simulink model "Channelizer_smoke"  (R2025a)
settings: Solver=VariableStepAuto  StartTime=0.0  StopTime=8359  RelTol=1e-3
PostLoadFcn:
  | gen_coeffs;
InitFcn:
  | gen_coeffs;
values from neighbouring files (symbols this model uses):
  coeff_matrix = zeros([num_fir_units, default_num_chan, fir_taps])    [coeffs_for_fir_units.m]    (also in gen_coeffs.m = squeeze(coeffs_for_fir_units(prototype_fir, config))')
undefined symbols (not defined in the file or in its folder): dspblkCoreblockFVToolHelper, es1, gcbh, S, vsva2488, xcvr1602
libraries: hdlBasic x27, dspsrcs4 x17, hdlDSPIP x1, vmcUtilities x1
settings Model: Creator=nanumolu  LastModifiedBy=robg

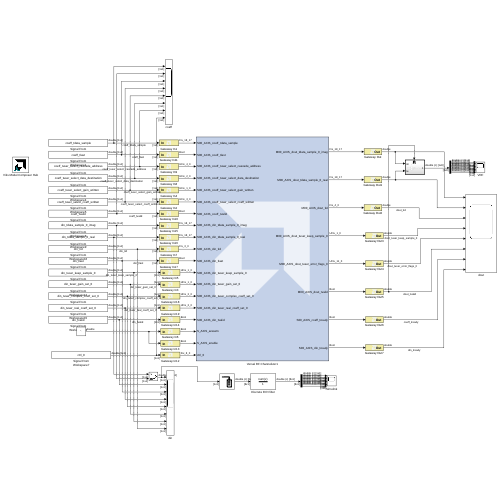
[thumbnail: Simulink's stored preview of the top-level diagram]
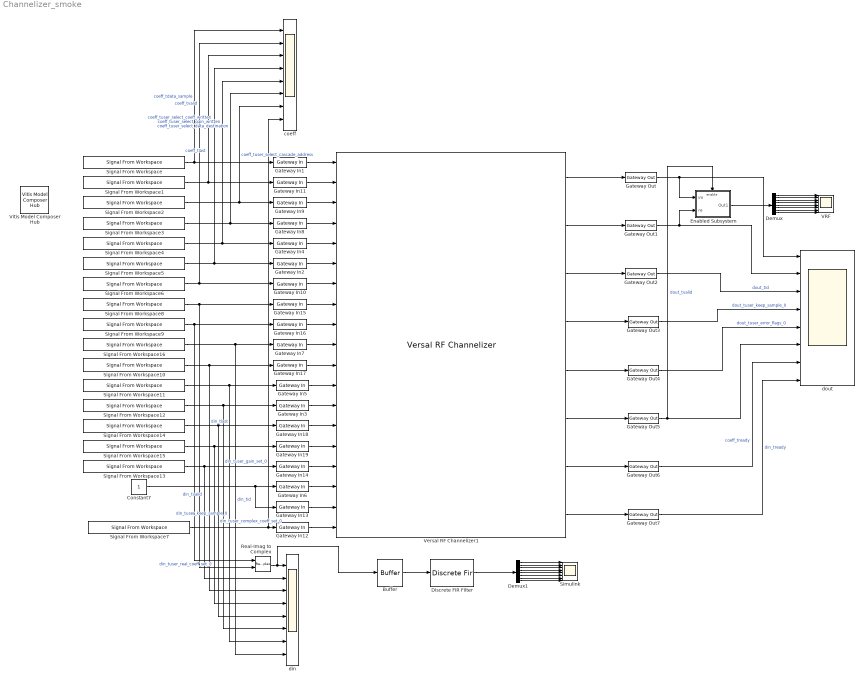
== system Channelizer_smoke ==
  Buffer : Buffer  N=8  OutputFrames=off
  Constant7 : Constant
  Demux : Demux  Outputs=8
  Demux1 : Demux  Outputs=8
  Discrete FIR Filter : DiscreteFir  LoadFcn=dspblkCoreblockFVToolHelper(gcbh,'load');  Coefficients=coeff_matrix(:,1)'  InputProcessing=Columns as channels (frame based)
      settings: CopyFcn=dspblkCoreblockFVToolHelper(gcbh,'copy');  DeleteFcn=dspblkCoreblockFVToolHelper(gcbh,'close');  ModelCloseFcn=dspblkCoreblockFVToolHelper(gcbh,'close');  PreSaveFcn=dspblkCoreblockFVToolHelper(gcbh,'presave');  PostSaveFcn=dspblkCoreblockFVToolHelper(gcbh,'postsave');  CloseFcn=dspblkCoreblockFVToolHelper(gcbh,'close');
  Enabled Subsystem : Subsystem  TreatAsAtomicUnit=on
  Gateway In1 : hdlBasic/Gateway In  gui_display_data_type=Fixed-point  arith_type=Signed (2's comp)  n_bits=18  bin_pt=17  preci_type=Single  exp_width=8  frac_width=24  rows=1  columns=1  quantization="Round  (unbiased: +/- Inf)"  overflow=Saturate  period=1  UseAsADC=off  ADCChannel='1'  interface=None  automatic_assignment=on  address_offset=hex2dec('00')  intf_name=''  intf_description=''  default_value=0  timing_constraint=None  locs_specified=off  LOCs={}  io_standard={}  inherit_from_input=off  hdl_port=on  XmcBlockStatus=1  maskContainerNames=group4  block_type=gatewayin  block_config=sysgen:gateway_in_config  block_width_w=590  block_height_w=620  block_width=640  block_height=850
  Gateway In{6,10..11,13..14,17} (6 alike) : hdlBasic/Gateway In  gui_display_data_type=Boolean  arith_type=Boolean  n_bits=16  bin_pt=14  preci_type=Single  exp_width=8  frac_width=24  rows=1  columns=1  quantization="Round  (unbiased: +/- Inf)"  overflow=Saturate  period=1  UseAsADC=off  ADCChannel='1'  interface=None  automatic_assignment=on  address_offset=hex2dec('00')  intf_name=''  intf_description=''  default_value=0  timing_constraint=None  locs_specified=off  LOCs={}  io_standard={}  inherit_from_input=off  hdl_port=on  XmcBlockStatus=1  maskContainerNames=group4  block_type=gatewayin  block_config=sysgen:gateway_in_config  block_width_w=590  block_height_w=620  block_width=640  block_height=850
  Gateway In12 : hdlBasic/Gateway In  gui_display_data_type=Fixed-point  arith_type=Signed (2's comp)  n_bits=8  bin_pt=0  preci_type=Single  exp_width=8  frac_width=24  rows=1  columns=1  quantization="Round  (unbiased: +/- Inf)"  overflow=Saturate  period=1  UseAsADC=off  ADCChannel='1'  interface=None  automatic_assignment=on  address_offset=hex2dec('00')  intf_name=''  intf_description=''  default_value=0  timing_constraint=None  locs_specified=off  LOCs={}  io_standard={}  inherit_from_input=off  hdl_port=on  XmcBlockStatus=1  maskContainerNames=group4  block_type=gatewayin  block_config=sysgen:gateway_in_config  block_width_w=590  block_height_w=620  block_width=640  block_height=850
  Gateway In15 : hdlBasic/Gateway In  gui_display_data_type=Fixed-point  arith_type=Signed (2's comp)  n_bits=18  bin_pt=17  preci_type=Single  exp_width=8  frac_width=24  rows=1  columns=1  quantization="Round  (unbiased: +/- Inf)"  overflow=Saturate  period=1  UseAsADC=off  ADCChannel='1'  interface=None  automatic_assignment=on  address_offset=hex2dec('00')  intf_name=''  intf_description=''  default_value=0  timing_constraint=None  locs_specified=off  LOCs={}  io_standard={}  inherit_from_input=off  hdl_port=on  XmcBlockStatus=1  maskContainerNames=group4  block_type=gatewayin  block_config=sysgen:gateway_in_config  block_width_w=590  block_height_w=620  block_width=640  block_height=850
  Gateway In16 : hdlBasic/Gateway In  gui_display_data_type=Fixed-point  arith_type=Signed (2's comp)  n_bits=18  bin_pt=17  preci_type=Single  exp_width=8  frac_width=24  rows=1  columns=1  quantization="Round  (unbiased: +/- Inf)"  overflow=Saturate  period=1  UseAsADC=off  ADCChannel='1'  interface=None  automatic_assignment=on  address_offset=hex2dec('00')  intf_name=''  intf_description=''  default_value=0  timing_constraint=None  locs_specified=off  LOCs={}  io_standard={}  inherit_from_input=off  hdl_port=on  XmcBlockStatus=1  maskContainerNames=group4  block_type=gatewayin  block_config=sysgen:gateway_in_config  block_width_w=590  block_height_w=620  block_width=640  block_height=850
  Gateway In18 : hdlBasic/Gateway In  gui_display_data_type=Fixed-point  arith_type=Unsigned  n_bits=3  bin_pt=0  preci_type=Single  exp_width=8  frac_width=24  rows=1  columns=1  quantization="Round  (unbiased: +/- Inf)"  overflow=Saturate  period=1  UseAsADC=off  ADCChannel='1'  interface=None  automatic_assignment=on  address_offset=hex2dec('00')  intf_name=''  intf_description=''  default_value=0  timing_constraint=None  locs_specified=off  LOCs={}  io_standard={}  inherit_from_input=off  hdl_port=on  XmcBlockStatus=1  maskContainerNames=group4  block_type=gatewayin  block_config=sysgen:gateway_in_config  block_width_w=590  block_height_w=620  block_width=640  block_height=850
  Gateway In19 : hdlBasic/Gateway In  gui_display_data_type=Fixed-point  arith_type=Unsigned  n_bits=3  bin_pt=0  preci_type=Single  exp_width=8  frac_width=24  rows=1  columns=1  quantization="Round  (unbiased: +/- Inf)"  overflow=Saturate  period=1  UseAsADC=off  ADCChannel='1'  interface=None  automatic_assignment=on  address_offset=hex2dec('00')  intf_name=''  intf_description=''  default_value=0  timing_constraint=None  locs_specified=off  LOCs={}  io_standard={}  inherit_from_input=off  hdl_port=on  XmcBlockStatus=1  maskContainerNames=group4  block_type=gatewayin  block_config=sysgen:gateway_in_config  block_width_w=590  block_height_w=620  block_width=640  block_height=850
  Gateway In2 : hdlBasic/Gateway In  gui_display_data_type=Fixed-point  arith_type=Unsigned  n_bits=3  bin_pt=0  preci_type=Single  exp_width=8  frac_width=24  rows=1  columns=1  quantization="Round  (unbiased: +/- Inf)"  overflow=Saturate  period=1  UseAsADC=off  ADCChannel='1'  interface=None  automatic_assignment=on  address_offset=hex2dec('00')  intf_name=''  intf_description=''  default_value=0  timing_constraint=None  locs_specified=off  LOCs={}  io_standard={}  inherit_from_input=off  hdl_port=on  XmcBlockStatus=1  maskContainerNames=group4  block_type=gatewayin  block_config=sysgen:gateway_in_config  block_width_w=590  block_height_w=620  block_width=640  block_height=850
  Gateway In3 : hdlBasic/Gateway In  gui_display_data_type=Fixed-point  arith_type=Unsigned  n_bits=1  bin_pt=0  preci_type=Single  exp_width=8  frac_width=24  rows=1  columns=1  quantization="Round  (unbiased: +/- Inf)"  overflow=Saturate  period=1  UseAsADC=off  ADCChannel='1'  interface=None  automatic_assignment=on  address_offset=hex2dec('00')  intf_name=''  intf_description=''  default_value=0  timing_constraint=None  locs_specified=off  LOCs={}  io_standard={}  inherit_from_input=off  hdl_port=on  XmcBlockStatus=1  maskContainerNames=group4  block_type=gatewayin  block_config=sysgen:gateway_in_config  block_width_w=590  block_height_w=620  block_width=640  block_height=850
  Gateway In4 : hdlBasic/Gateway In  gui_display_data_type=Fixed-point  arith_type=Unsigned  n_bits=1  bin_pt=0  preci_type=Single  exp_width=8  frac_width=24  rows=1  columns=1  quantization="Round  (unbiased: +/- Inf)"  overflow=Saturate  period=1  UseAsADC=off  ADCChannel='1'  interface=None  automatic_assignment=on  address_offset=hex2dec('00')  intf_name=''  intf_description=''  default_value=0  timing_constraint=None  locs_specified=off  LOCs={}  io_standard={}  inherit_from_input=off  hdl_port=on  XmcBlockStatus=1  maskContainerNames=group4  block_type=gatewayin  block_config=sysgen:gateway_in_config  block_width_w=590  block_height_w=620  block_width=640  block_height=850
  Gateway In5 : hdlBasic/Gateway In  gui_display_data_type=Fixed-point  arith_type=Unsigned  n_bits=1  bin_pt=0  preci_type=Single  exp_width=8  frac_width=24  rows=1  columns=1  quantization="Round  (unbiased: +/- Inf)"  overflow=Saturate  period=1  UseAsADC=off  ADCChannel='1'  interface=None  automatic_assignment=on  address_offset=hex2dec('00')  intf_name=''  intf_description=''  default_value=0  timing_constraint=None  locs_specified=off  LOCs={}  io_standard={}  inherit_from_input=off  hdl_port=on  XmcBlockStatus=1  maskContainerNames=group4  block_type=gatewayin  block_config=sysgen:gateway_in_config  block_width_w=590  block_height_w=620  block_width=640  block_height=850
  Gateway In7 : hdlBasic/Gateway In  gui_display_data_type=Fixed-point  arith_type=Signed (2's comp)  n_bits=3  bin_pt=0  preci_type=Single  exp_width=8  frac_width=24  rows=1  columns=1  quantization="Round  (unbiased: +/- Inf)"  overflow=Saturate  period=1  UseAsADC=off  ADCChannel='1'  interface=None  automatic_assignment=on  address_offset=hex2dec('00')  intf_name=''  intf_description=''  default_value=0  timing_constraint=None  locs_specified=off  LOCs={}  io_standard={}  inherit_from_input=off  hdl_port=on  XmcBlockStatus=1  maskContainerNames=group4  block_type=gatewayin  block_config=sysgen:gateway_in_config  block_width_w=590  block_height_w=620  block_width=640  block_height=850
  Gateway In8 : hdlBasic/Gateway In  gui_display_data_type=Fixed-point  arith_type=Unsigned  n_bits=2  bin_pt=0  preci_type=Single  exp_width=8  frac_width=24  rows=1  columns=1  quantization="Round  (unbiased: +/- Inf)"  overflow=Saturate  period=1  UseAsADC=off  ADCChannel='1'  interface=None  automatic_assignment=on  address_offset=hex2dec('00')  intf_name=''  intf_description=''  default_value=0  timing_constraint=None  locs_specified=off  LOCs={}  io_standard={}  inherit_from_input=off  hdl_port=on  XmcBlockStatus=1  maskContainerNames=group4  block_type=gatewayin  block_config=sysgen:gateway_in_config  block_width_w=590  block_height_w=620  block_width=640  block_height=850
  Gateway In9 : hdlBasic/Gateway In  gui_display_data_type=Fixed-point  arith_type=Unsigned  n_bits=4  bin_pt=0  preci_type=Single  exp_width=8  frac_width=24  rows=1  columns=1  quantization="Round  (unbiased: +/- Inf)"  overflow=Saturate  period=1  UseAsADC=off  ADCChannel='1'  interface=None  automatic_assignment=on  address_offset=hex2dec('00')  intf_name=''  intf_description=''  default_value=0  timing_constraint=None  locs_specified=off  LOCs={}  io_standard={}  inherit_from_input=off  hdl_port=on  XmcBlockStatus=1  maskContainerNames=group4  block_type=gatewayin  block_config=sysgen:gateway_in_config  block_width_w=590  block_height_w=620  block_width=640  block_height=850
  Gateway Out{,1..7} (8 alike) : hdlBasic/Gateway Out  inherit_from_input=off  bool_to_boolean=off  hdl_port=on  rows=1  columns=1  UseAsDAC=off  DACChannel='1'  interface=None  automatic_assignment=on  address_offset=hex2dec('00')  intf_name=''  intf_description=''  timing_constraint=None  locs_specified=off  LOCs={}  io_standard={}  XmcBlockStatus=1  maskContainerNames=group4  block_type=gatewayout  block_config=sysgen:gateway_out_config  block_width_w=590  block_height_w=620  block_width=620  block_height=750
  Real-Imag to Complex : RealImagToComplex
  Signal From Workspace : dspsrcs4/Signal From Workspace  X=coeff_tdata_sample  Ts=1  nsamps=1  OutputAfterFinalValue=Setting to zero  ignoreOrWarnInputAndFrameLengths=off  OutputFrames=off
  Signal From Workspace1 : dspsrcs4/Signal From Workspace  X=coeff_tlast  Ts=1  nsamps=1  OutputAfterFinalValue=Setting to zero  ignoreOrWarnInputAndFrameLengths=off  OutputFrames=off
  Signal From Workspace10 : dspsrcs4/Signal From Workspace  X=din_tlast  Ts=1  nsamps=1  OutputAfterFinalValue=Setting to zero  ignoreOrWarnInputAndFrameLengths=off  OutputFrames=off
  Signal From Workspace11 : dspsrcs4/Signal From Workspace  X=din_tuser_keep_sample_0  Ts=1  nsamps=1  OutputAfterFinalValue=Setting to zero  ignoreOrWarnInputAndFrameLengths=off  OutputFrames=off
  Signal From Workspace12 : dspsrcs4/Signal From Workspace  X=din_tuser_gain_set_0  Ts=1  nsamps=1  OutputAfterFinalValue=Setting to zero  ignoreOrWarnInputAndFrameLengths=off  OutputFrames=off
  Signal From Workspace13 : dspsrcs4/Signal From Workspace  X=din_tvalid  Ts=1  nsamps=1  OutputAfterFinalValue=Setting to zero  ignoreOrWarnInputAndFrameLengths=off  OutputFrames=off
  Signal From Workspace14 : dspsrcs4/Signal From Workspace  X=din_tuser_complex_coeff_set_0  Ts=1  nsamps=1  OutputAfterFinalValue=Setting to zero  ignoreOrWarnInputAndFrameLengths=off  OutputFrames=off
  Signal From Workspace15 : dspsrcs4/Signal From Workspace  X=din_tuser_real_coeff_set_0  Ts=1  nsamps=1  OutputAfterFinalValue=Setting to zero  ignoreOrWarnInputAndFrameLengths=off  OutputFrames=off
  Signal From Workspace16 : dspsrcs4/Signal From Workspace  X=din_tid  Ts=1  nsamps=1  OutputAfterFinalValue=Setting to zero  ignoreOrWarnInputAndFrameLengths=off  OutputFrames=off
  Signal From Workspace2 : dspsrcs4/Signal From Workspace  X=coeff_tuser_select_cascade_address  Ts=1  nsamps=1  OutputAfterFinalValue=Setting to zero  ignoreOrWarnInputAndFrameLengths=off  OutputFrames=off
  Signal From Workspace3 : dspsrcs4/Signal From Workspace  X=coeff_tuser_select_data_destination  Ts=1  nsamps=1  OutputAfterFinalValue=Setting to zero  ignoreOrWarnInputAndFrameLengths=off  OutputFrames=off
  Signal From Workspace4 : dspsrcs4/Signal From Workspace  X=coeff_tuser_select_gain_written  Ts=1  nsamps=1  OutputAfterFinalValue=Setting to zero  ignoreOrWarnInputAndFrameLengths=off  OutputFrames=off
  Signal From Workspace5 : dspsrcs4/Signal From Workspace  X=coeff_tuser_select_coeff_written  Ts=1  nsamps=1  OutputAfterFinalValue=Setting to zero  ignoreOrWarnInputAndFrameLengths=off  OutputFrames=off
  Signal From Workspace6 : dspsrcs4/Signal From Workspace  X=coeff_tvalid  Ts=1  nsamps=1  OutputAfterFinalValue=Setting to zero  ignoreOrWarnInputAndFrameLengths=off  OutputFrames=off
  Signal From Workspace7 : dspsrcs4/Signal From Workspace  X=ctrl_0  Ts=1  nsamps=1  OutputAfterFinalValue=Setting to zero  ignoreOrWarnInputAndFrameLengths=off  OutputFrames=off
  Signal From Workspace8 : dspsrcs4/Signal From Workspace  X=din_tdata_sample_0_imag  Ts=1  nsamps=1  OutputAfterFinalValue=Setting to zero  ignoreOrWarnInputAndFrameLengths=off  OutputFrames=off
  Signal From Workspace9 : dspsrcs4/Signal From Workspace  X=din_tdata_sample_0_real  Ts=1  nsamps=1  OutputAfterFinalValue=Setting to zero  ignoreOrWarnInputAndFrameLengths=off  OutputFrames=off
  Simulink : Scope  NumInputPorts=8
      settings: TimeUnits=Metric (based on Time Span)  ActiveDisplayYMinimum=-0.37489960244638232  ActiveDisplayYMaximum=0.37494511836079  YLabel=Amplitude  DataLoggingVariableName=ScopeData4
  VRF : Scope  NumInputPorts=8
      settings: TimeUnits=Metric (based on Time Span)  ActiveDisplayYMinimum=-0.0001049041748046875  ActiveDisplayYMaximum=0.0001049041748046875  YLabel=Amplitude  DataLoggingVariableName=ScopeData3
  Versal RF Channelizer1 : hdlDSPIP/Versal RF Channelizer  mode=FIR Filter  input_sample_rate=1  num_of_instances=1  fft_direction=FFT  fft_sync_on_tlast=off  fir_coeff_type=Real  fir_length=16  gain_en=off  events=off  coeff_casc_en=off  active_duty_cycle=25  toggle_rate=25  fir_unit_0_taps=16  fir_unit_1_taps=0  fir_unit_2_taps=0  fir_unit_3_taps=0  ip_name=Versal RF Channelizer  enable_all_ports=false  ip_version=1.1  dsptool_ready=false  ipcore_usecache=true  ipcore_useipmodelcache=true  wrapper_available=true  port_translation_map={ 'aclken' => 'en', 'aresetn' => 'rst' }  structural_sim=true  ipcore_do_not_force_period=true  oldconvolution_code_radix=Binary  XmcBlockStatus=1  maskContainerNames=tabcontainer1  block_type=vrf_channelizer_v1_1  block_config=sysgen:rodinimport_config
  Vitis Model Composer Hub : vmcUtilities/Vitis Model Composer Hub  Tag=genX  CodeGeneration=off  SubsystemName=DUT  BlockHierPath=Channalizer_smoke  CompilationType=HDLCompilation  SubsystemType=HDLNode  ExportTypeV2=HDL Netlist  StartColumn=1  NumberOfColumns=1  TargetDirectory=./netlist_chan_vlg  exportDesign=on  analyzeDesign=off  validateDesignOnHw=off  ExportType=AI Engines  IpVendor=xilinx.com  IpLibrary=hls  IpVersion=1.0  IpHWLanguage=Verilog  AieCompilerOptions={}  AieSimulatorOptions={}  CreateTestbench=on  TestbenchStackSize=10  RunRtlSim=off  RunCSim=off  RunAieSim=off  AieSimTimeout=50000  RunAieSimProfiling=off  LaunchVitisAnalyzer=off  PlotOutput=off  RunX86Sim=off  X86SimTimeout=10  GenHwImage=off  GenLibadfXo=on  GenHwValidationCode=off  PlatformType=Not Specified  HwSystemType=Baremetal  HwValidationTarget=hw  ProjDevice=xcvr1602-vsva2488-2MP-e-S-es1  ProjDevicePart=xcvr1602-vsva2488-2MP-e-S-es1  AIEType=AIE  SamplePeriod=-1  ClockFrequency=200  DataPathParallelism=1  xilinxfamily=versalairfes1  part=xcvr1602  speed=-2MP-e-S-es1  package=vsva2488  directory=./netlist/ip/DUT/src  testbench=off  incr_netlist=off  synthesis_tool=Vivado  clock_wrapper=Clock Enables  dbl_ovrd=According to Block Masks  dcm_input_clock_period=10  sysclk_period=10  simulink_period=1  eval_field=0  IPInfoJsonString="{\"DUTSubsystemName\":\"Channalizer_smoke\",\"HDLSubsystem\":{\"SubsystemName\":\"Channalizer_smoke\",\"IPName\":\"Copy_of_hamilton_vrf_fft\",\"IPLibrary\":\"VMC\",\"IPVendor\":\"User Company\",\"IPVersion\":\"1.0\",\"TargetDirectory\":\"./netlist_chan_vlg\",\"SubsystemDir\":\"./netlist_chan_vlg/ip/Channalizer_smoke\",\"FreqHz\":\"100000000\"},\"SubsystemTag\":\"HDLNode\"}"  LogFileName=/proj/dsv_xhd/ravalib/Head/Tests/REL/2025.1/dsv/modelcomposer/hdl/regression/channelizer/smoke/netlist_chan_vlg/model_composer.log  NThreads=4  IPConfigFile=/tmp/vmctmp-10364637636032824832/Channalizer_smoke_ipconfig.json
  coeff : Scope  NumInputPorts=8
      settings: TimeUnits=Metric (based on Time Span)  ActiveDisplayYMinimum=-0.28314140423786416  ActiveDisplayYMaximum=1.187124788118022  YLabel=Amplitude
  din : Scope  NumInputPorts=8
      settings: TimeUnits=Metric (based on Time Span)  ActiveDisplayYMinimum=-0.17153741308923837  ActiveDisplayYMaximum=0.35239304589880421  YLabel=Amplitude  DataLoggingVariableName=ScopeData2
  dout : Scope  NumInputPorts=8
      settings: ActiveDisplayYMinimum=-1  ActiveDisplayYMaximum=1
  wires:
  Gateway Out/1 -> Enabled Subsystem/1(im), dout/1
  Gateway Out1/1 -> Enabled Subsystem/2(re), dout/2
  Gateway Out2/1 -> dout/3  "dout_tid"
  Gateway Out3/1 -> dout/4  "dout_tuser_keep_sample_0"
  Gateway Out4/1 -> dout/5  "dout_tuser_error_flags_0"
  Gateway Out5/1 -> Enabled Subsystem/Enable, dout/6  "dout_tvalid"
  Gateway Out6/1 -> dout/7  "coeff_tready"
  Gateway Out7/1 -> dout/8  "din_tready"
  Constant7/1 -> Gateway In13/1, Gateway In6/1
  Versal RF Channelizer1/8 -> Gateway Out7/1
  Versal RF Channelizer1/1 -> Gateway Out/1
  Versal RF Channelizer1/3 -> Gateway Out2/1
  Versal RF Channelizer1/5 -> Gateway Out4/1
  Versal RF Channelizer1/7 -> Gateway Out6/1
  Versal RF Channelizer1/6 -> Gateway Out5/1
  Versal RF Channelizer1/4 -> Gateway Out3/1
  Versal RF Channelizer1/2 -> Gateway Out1/1
  Signal From Workspace/1 -> coeff/1, Gateway In1/1  "coeff_tdata_sample"
  Gateway In1/1 -> Versal RF Channelizer1/1
  Signal From Workspace5/1 -> coeff/4, Gateway In2/1  "coeff_tuser_select_coeff_written"
  Gateway In2/1 -> Versal RF Channelizer1/6
  Signal From Workspace4/1 -> coeff/5, Gateway In4/1  "coeff_tuser_select_gain_written"
  Gateway In4/1 -> Versal RF Channelizer1/5
  Signal From Workspace2/1 -> coeff/7, Gateway In9/1  "coeff_tuser_select_cascade_address"
  Gateway In9/1 -> Versal RF Channelizer1/3
  Signal From Workspace3/1 -> coeff/6, Gateway In8/1  "coeff_tuser_select_data_destination"
  Gateway In8/1 -> Versal RF Channelizer1/4
  Signal From Workspace6/1 -> coeff/2, Gateway In10/1  "coeff_tvalid"
  Gateway In10/1 -> Versal RF Channelizer1/7
  Signal From Workspace1/1 -> coeff/3, Gateway In11/1  "coeff_tlast"
  Gateway In11/1 -> Versal RF Channelizer1/2
  Signal From Workspace7/1 -> coeff/8, Gateway In12/1
  Gateway In15/1 -> Versal RF Channelizer1/8
  Gateway In16/1 -> Versal RF Channelizer1/9
  Signal From Workspace8/1 -> Real-Imag to Complex/2, Gateway In15/1
  Signal From Workspace9/1 -> Real-Imag to Complex/1, Gateway In16/1
  Signal From Workspace10/1 -> din/3, Gateway In17/1  "din_tlast"
  Signal From Workspace11/1 -> din/7, Gateway In5/1  "din_tuser_keep_sample_0"
  Signal From Workspace12/1 -> din/6, Gateway In3/1  "din_tuser_gain_set_0"
  Signal From Workspace13/1 -> din/2, Gateway In14/1  "din_tvalid"
  Signal From Workspace14/1 -> din/5, Gateway In18/1  "din_tuser_complex_coeff_set_0"
  Signal From Workspace15/1 -> din/4, Gateway In19/1  "din_tuser_real_coeff_set_0"
  Real-Imag to Complex/1 -> Buffer/1, din/1
  Gateway In7/1 -> Versal RF Channelizer1/10
  Gateway In17/1 -> Versal RF Channelizer1/11
  Gateway In5/1 -> Versal RF Channelizer1/12
  Gateway In3/1 -> Versal RF Channelizer1/13
  Gateway In18/1 -> Versal RF Channelizer1/14
  Gateway In19/1 -> Versal RF Channelizer1/15
  Gateway In14/1 -> Versal RF Channelizer1/16
  Gateway In6/1 -> Versal RF Channelizer1/17
  Gateway In13/1 -> Versal RF Channelizer1/18
  Gateway In12/1 -> Versal RF Channelizer1/19
  Signal From Workspace16/1 -> Gateway In7/1, din/8  "din_tid"
  Enabled Subsystem/1(Out1) -> Demux/1
  Buffer/1 -> Discrete FIR Filter/1
  Demux/1 -> VRF/1
  Demux/2 -> VRF/2
  Demux/3 -> VRF/3
  Demux/4 -> VRF/4
  Demux/5 -> VRF/5
  Demux/6 -> VRF/6
  Demux/7 -> VRF/7
  Demux/8 -> VRF/8
  Demux1/8 -> Simulink/8
  Demux1/7 -> Simulink/7
  Demux1/6 -> Simulink/6
  Demux1/5 -> Simulink/5
  Demux1/4 -> Simulink/4
  Demux1/3 -> Simulink/3
  Demux1/2 -> Simulink/2
  Demux1/1 -> Simulink/1
  Discrete FIR Filter/1 -> Demux1/1

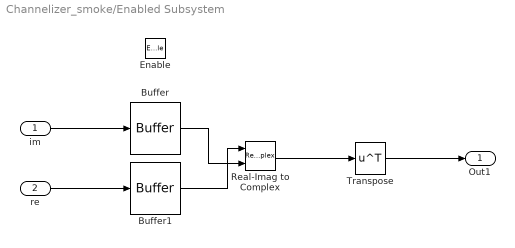
== system Channelizer_smoke/Enabled Subsystem ==
  im : Inport
  re : Inport  Port=2
  Enable : EnablePort
  Buffer : Buffer  N=8  OutputFrames=off
  Buffer1 : Buffer  N=8  OutputFrames=off
  Real-Imag to Complex : RealImagToComplex
  Transpose : Math  Operator=transpose
  Out1 : Outport
  wires:
  re/1 -> Buffer1/1
  im/1 -> Buffer/1
  Buffer/1 -> Real-Imag to Complex/2
  Buffer1/1 -> Real-Imag to Complex/1
  Real-Imag to Complex/1 -> Transpose/1
  Transpose/1 -> Out1/1
